simulink model "cip_sim"  (R2021a)
settings: Solver=VariableStepAuto  StartTime=0.0  StopTime=30  MaxStep=0.01  RelTol=1e-3
undefined symbols (not defined in the file or in its folder): A, B, dF_amp, dF_tf, G_icare, K_gms, r, x0
libraries: cstblocks x1
settings Model: Creator=Brent  LastModifiedBy=Brent
settings SolverCC: AlgebraicLoopSolver=TrustRegion
settings DebuggingCC: SFMachineParentedDataDiag=warning

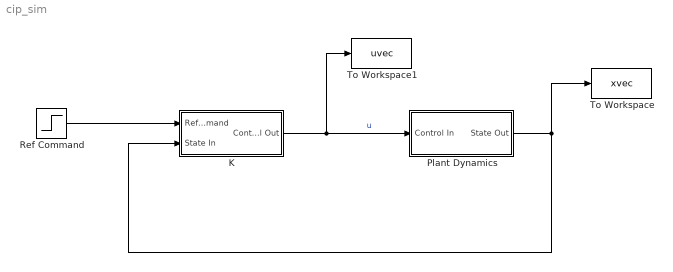
== system cip_sim ==
  K : Subsystem
  Plant Dynamics : Subsystem
  Ref Command : Step  Time=0  After=r  SampleTime=0
  To Workspace : ToWorkspace  VariableName=xvec  SaveFormat=Timeseries  SampleTime=-1
  To Workspace1 : ToWorkspace  VariableName=uvec  SaveFormat=Timeseries  SampleTime=-1
  wires:
  Plant Dynamics/1(State Out) -> K/2(State In), To Workspace/1
  K/1(Control Out) -> To Workspace1/1, Plant Dynamics/1(Control In)  "u"
  Ref Command/1 -> K/1(Reference Command)

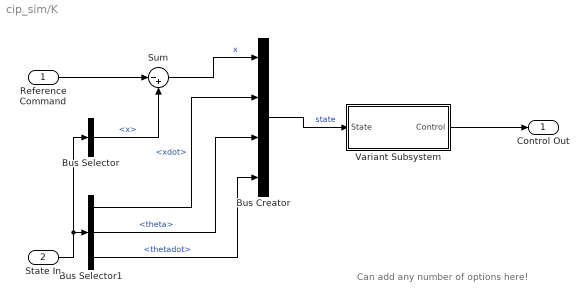
== system cip_sim/K ==
  note: Can add any number of options here!
  Reference Command : Inport
  State In : Inport  Port=2
  Bus Creator : BusCreator  Inputs=4
  Bus Selector : BusSelector  OutputSignals=x
  Bus Selector1 : BusSelector  OutputSignals=xdot,theta,thetadot
  Sum : Sum  Inputs=|-+
  Variant Subsystem : Subsystem  Variant=on
  Control Out : Outport
  wires:
  State In/1 -> Bus Selector/1, Bus Selector1/1
  Reference Command/1 -> Sum/1
  Bus Selector/1 -> Sum/2  "<x>"
  Sum/1 -> Bus Creator/1  "x"
  Bus Selector1/1 -> Bus Creator/2  "<xdot>"
  Bus Selector1/2 -> Bus Creator/3  "<theta>"
  Bus Selector1/3 -> Bus Creator/4  "<thetadot>"
  Bus Creator/1 -> Variant Subsystem/1(State)  "state"
  Variant Subsystem/1(Control) -> Control Out/1

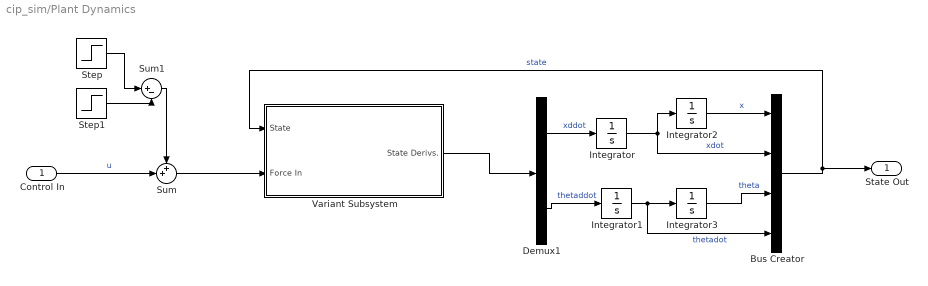
== system cip_sim/Plant Dynamics ==
  Control In : Inport
  Bus Creator : BusCreator  Inputs=4
  Demux1 : Demux  Outputs=2
  Integrator : Integrator  InitialCondition=x0(2)
  Integrator1 : Integrator  InitialCondition=x0(4)
  Integrator2 : Integrator  InitialCondition=x0(1)
  Integrator3 : Integrator  InitialCondition=x0(3)
  Step : Step  Time=0  After=dF_amp  SampleTime=0
  Step1 : Step  Time=dF_tf  After=dF_amp  SampleTime=0
  Sum : Sum  Inputs=++|
  Sum1 : Sum  Inputs=|+-
  Variant Subsystem : Subsystem  Variant=on
  State Out : Outport  VectorParamsAs1DForOutWhenUnconnected=off
  wires:
  Integrator/1 -> Bus Creator/2, Integrator2/1  "xdot"
  Demux1/1 -> Integrator/1  "xddot"
  Bus Creator/1 -> Variant Subsystem/1(State), State Out/1  "state"
  Control In/1 -> Sum/2  "u"
  Demux1/2 -> Integrator1/1  "thetaddot"
  Integrator2/1 -> Bus Creator/1  "x"
  Integrator1/1 -> Bus Creator/4, Integrator3/1  "thetadot"
  Integrator3/1 -> Bus Creator/3  "theta"
  Variant Subsystem/1(State Derivs.) -> Demux1/1
  Step/1 -> Sum1/1
  Sum/1 -> Variant Subsystem/2(Force In)
  Step1/1 -> Sum1/2
  Sum1/1 -> Sum/1

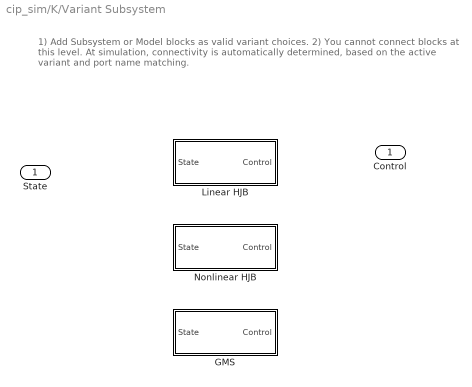
== system cip_sim/K/Variant Subsystem ==
  note: 1) Add Subsystem or Model blocks as valid variant choices.
      | 2) You cannot connect blocks at this level. At simulation, connectivity is automatically
      | determined, based on the active variant and port name matching.
  State : Inport
  GMS : Subsystem  VariantControl=v_gms
  Linear HJB : Subsystem  VariantControl=v_lin_hjb
  Nonlinear HJB : Subsystem  VariantControl=v_nonlin_hjb
  Control : Outport

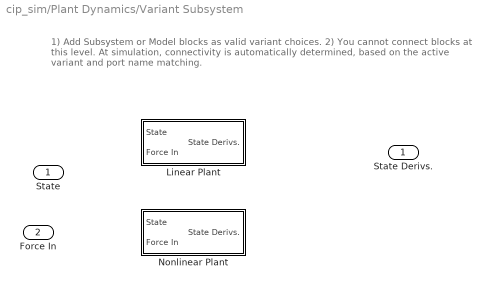
== system cip_sim/Plant Dynamics/Variant Subsystem ==
  note: 1) Add Subsystem or Model blocks as valid variant choices.
      | 2) You cannot connect blocks at this level. At simulation, connectivity is automatically
      | determined, based on the active variant and port name matching.
  State : Inport
  Force In : Inport  Port=2
  Linear Plant : Subsystem  VariantControl=v_linear_plant
  Nonlinear Plant : Subsystem  VariantControl=v_nonlinear_plant
  State Derivs. : Outport

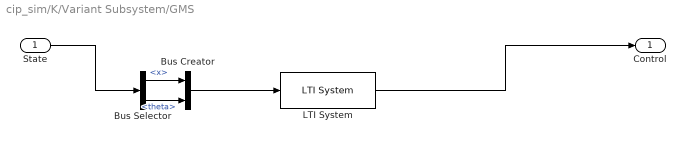
== system cip_sim/K/Variant Subsystem/GMS ==
  State : Inport
  Bus Creator : BusCreator  Inputs=2
  Bus Selector : BusSelector  OutputSignals=x,theta
  LTI System : cstblocks/LTI System  sys=-K_gms  IC=[]
  Control : Outport
  wires:
  LTI System/1 -> Control/1
  Bus Creator/1 -> LTI System/1
  State/1 -> Bus Selector/1
  Bus Selector/1 -> Bus Creator/1  "<x>"
  Bus Selector/2 -> Bus Creator/2  "<theta>"

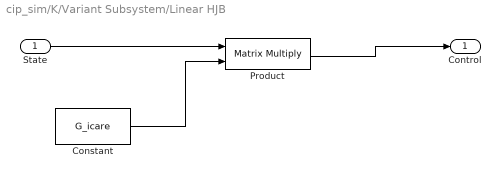
== system cip_sim/K/Variant Subsystem/Linear HJB ==
  State : Inport
  Constant : Constant  Value=G_icare
  Product : Product  Multiplication=Matrix(*)
  Control : Outport
  wires:
  State/1 -> Product/1
  Product/1 -> Control/1
  Constant/1 -> Product/2

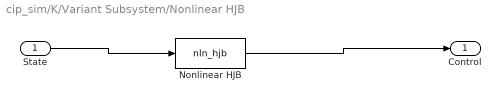
== system cip_sim/K/Variant Subsystem/Nonlinear HJB ==
  State : Inport
  Nonlinear HJB : MATLABFcn  MATLABFcn=nln_hjb
  Control : Outport
  wires:
  Nonlinear HJB/1 -> Control/1
  State/1 -> Nonlinear HJB/1

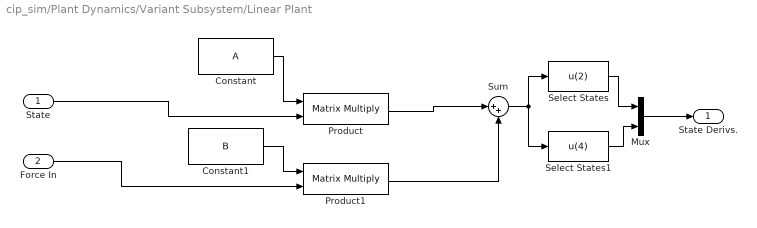
== system cip_sim/Plant Dynamics/Variant Subsystem/Linear Plant ==
  State : Inport
  Force In : Inport  Port=2
  Constant : Constant  Value=A
  Constant1 : Constant  Value=B
  Mux : Mux  Inputs=2
  Product : Product  Multiplication=Matrix(*)
  Product1 : Product  Multiplication=Matrix(*)
  Select States : Fcn  Expr=u(2)
  Select States1 : Fcn  Expr=u(4)
  Sum : Sum  Inputs=|++
  State Derivs. : Outport
  wires:
  Select States/1 -> Mux/1
  Select States1/1 -> Mux/2
  Constant1/1 -> Product1/1
  Mux/1 -> State Derivs./1
  Sum/1 -> Select States/1, Select States1/1
  State/1 -> Product/2
  Product1/1 -> Sum/2
  Constant/1 -> Product/1
  Force In/1 -> Product1/2
  Product/1 -> Sum/1

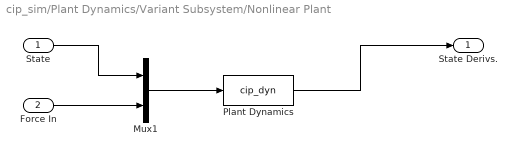
== system cip_sim/Plant Dynamics/Variant Subsystem/Nonlinear Plant ==
  State : Inport
  Force In : Inport  Port=2
  Mux1 : Mux  Inputs=2
  Plant Dynamics : MATLABFcn  MATLABFcn=cip_dyn
  State Derivs. : Outport
  wires:
  Mux1/1 -> Plant Dynamics/1
  Force In/1 -> Mux1/2
  State/1 -> Mux1/1
  Plant Dynamics/1 -> State Derivs./1
